simulink model "event_based_v1"  (R2018b)
settings: Solver=FixedStepAuto  StartTime=0.0  StopTime=150  FixedStep=0.01  RelTol=1e-3
undefined symbols (not defined in the file or in its folder): theta01, x01, y01
settings Model: Creator=root  LastModifiedBy=root

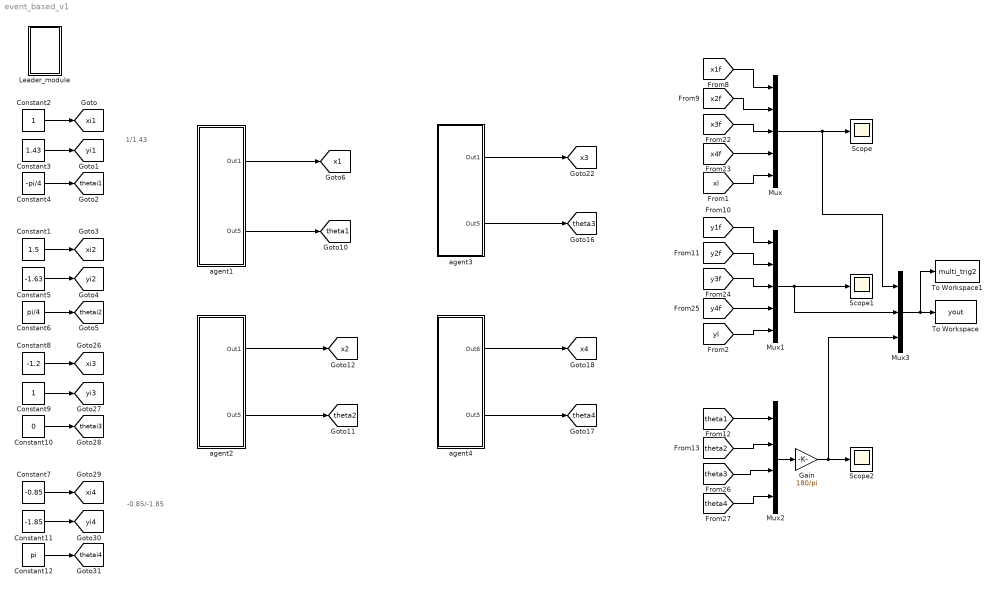
== system event_based_v1 ==
  note: 1/1.43
  note: -0.85/-1.85
  Constant1 : Constant  Value=1.5
  Constant10 : Constant  Value=0
  Constant11 : Constant  Value=-1.85
  Constant12 : Constant  Value=pi
  Constant2 : Constant
  Constant3 : Constant  Value=1.43
  Constant4 : Constant  Value=-pi/4
  Constant5 : Constant  Value=-1.63
  Constant6 : Constant  Value=pi/4
  Constant7 : Constant  Value=-0.85
  Constant8 : Constant  Value=-1.2
  Constant9 : Constant
  Gain : Gain  Gain=180/pi
  Leader_module : Subsystem
  Mux : Mux  Inputs=5
  Mux1 : Mux  Inputs=5
  Mux2 : Mux
  Mux3 : Mux  Inputs=3
  Scope : Scope
  Scope1 : Scope
  Scope2 : Scope
  To Workspace : ToWorkspace  VariableName=yout  SampleTime=-1
      settings: Save2DSignal=2-D array (concatenate along first dimension)
  To Workspace1 : ToWorkspace  VariableName=multi_trig2  SaveFormat=Structure With Time  SampleTime=-1
  agent1 : Subsystem
  agent2 : Subsystem
  agent3 : Subsystem
  agent4 : Subsystem
  tag scope: theta1=global, theta2=global, theta3=global, theta4=global, thetai1=global, thetai2=global, thetai3=global, thetai4=global, x1=global, x2=global, x3=global, x4=global, xi1=global, xi2=global, xi3=global, xi4=global, yi1=global, yi2=global, yi3=global, yi4=global
  wires:
  Mux3/1 -> To Workspace/1, To Workspace1/1
  Mux2/1 -> Gain/1
  [theta4] -> Mux2/4
  [theta3] -> Mux2/3
  [theta2] -> Mux2/2
  Mux1/1 -> Scope1/1, Mux3/2
  [y4f] -> Mux1/4
  [y3f] -> Mux1/3
  [y2f] -> Mux1/2
  [x4f] -> Mux/4
  [x3f] -> Mux/3
  Constant9/1 -> [yi3]
  Constant10/1 -> [thetai3]
  Constant8/1 -> [xi3]
  Constant7/1 -> [xi4]
  Constant12/1 -> [thetai4]
  Constant11/1 -> [yi4]
  agent3/2(Out5) -> [theta3]
  agent4/2(Out5) -> [theta4]
  Gain/1 -> Scope2/1, Mux3/3
  [theta1] -> Mux2/1
  Mux/1 -> Mux3/1, Scope/1
  [y1f] -> Mux1/1
  [x2f] -> Mux/2
  [x1f] -> Mux/1
  agent2/2(Out5) -> [theta2]
  agent1/2(Out5) -> [theta1]
  Constant5/1 -> [yi2]
  Constant6/1 -> [thetai2]
  Constant1/1 -> [xi2]
  Constant2/1 -> [xi1]
  Constant4/1 -> [thetai1]
  Constant3/1 -> [yi1]
  [xl] -> Mux/5
  [yl] -> Mux1/5
  agent1/1(Out1) -> [x1]
  agent2/1(Out1) -> [x2]
  agent3/1(Out1) -> [x3]
  agent4/1(Out6) -> [x4]

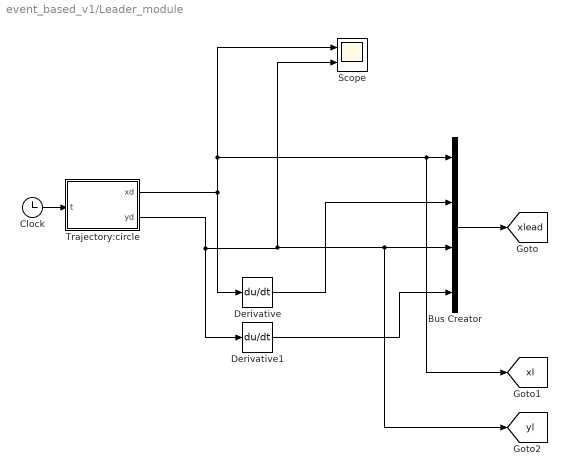
== system event_based_v1/Leader_module ==
  Bus Creator : BusCreator  Inputs=4
  Clock : Clock
  Derivative : Derivative
  Derivative1 : Derivative
  Scope : Scope  NumInputPorts=2
  Trajectory:circle : MATLAB Function  TreatAsAtomicUnit=on
  tag scope: xl=global, xlead=global, yl=global
  wires:
  Trajectory:circle/2(yd) -> [yl], Bus Creator/3, Scope/2, Derivative1/1
  Trajectory:circle/1(xd) -> Scope/1, [xl], Bus Creator/1, Derivative/1
  Clock/1 -> Trajectory:circle/1(t)
  Bus Creator/1 -> [xlead]
  Derivative/1 -> Bus Creator/2
  Derivative1/1 -> Bus Creator/4

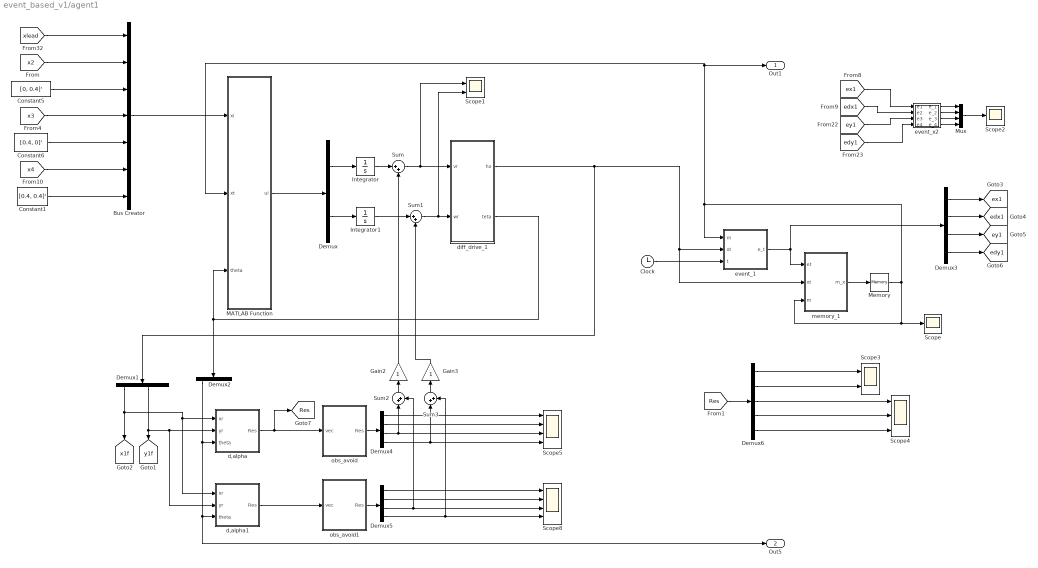
== system event_based_v1/agent1 ==
  Bus Creator : BusCreator  Inputs=7
  Clock : Clock
  Constant1 : Constant  Value=[0.4, 0.4]'
  Constant5 : Constant  Value=[0, 0.4]'
  Constant6 : Constant  Value=[0.4, 0]'
  Demux : Demux  Outputs=2
  Demux{1,3..5} (4 alike) : Demux
  Demux2 : Demux  Outputs=3
  Demux6 : Demux  Outputs=5
  Gain2 : Gain
  Gain3 : Gain
  Integrator : Integrator
  Integrator1 : Integrator
  MATLAB Function : MATLAB Function  TreatAsAtomicUnit=on
  Memory : Memory  InitialCondition=[0 0 0 0]'
  Mux : Mux
  Scope : Scope
  Scope1 : Scope  NumInputPorts=2
  Scope2 : Scope
  Scope3 : Scope  NumInputPorts=2
  Scope4 : Scope  NumInputPorts=3
  Scope5 : Scope  NumInputPorts=4
  Scope8 : Scope  NumInputPorts=4
  Sum{,1..3} (4 alike) : Sum  Inputs=|++
  d,alpha : MATLAB Function  TreatAsAtomicUnit=on
  d,alpha1 : MATLAB Function  TreatAsAtomicUnit=on
  diff_drive_1 : Subsystem  mask{base=0.078, base_error=2.5, radius=0.029, radius_error=6.9, omega_max=260}
      mask prompts: base_error "Base error in percent"; radius_error "Radius error in percent"; omega_max "Wheel Max Velocity"
  event_1 : MATLAB Function  TreatAsAtomicUnit=on
  event_x2 : MATLAB Function  TreatAsAtomicUnit=on
  memory_1 : MATLAB Function  TreatAsAtomicUnit=on
  "obs_avoid " : MATLAB Function  TreatAsAtomicUnit=on
  obs_avoid1 : MATLAB Function  TreatAsAtomicUnit=on
  Out1 : Outport
  Out5 : Outport  Port=2
  tag scope: Res=global, edx1=global, edy1=global, ex1=global, ey1=global, x1f=global, y1f=global
  wires:
  Sum3/1 -> Gain3/1
  Sum2/1 -> Gain2/1
  Gain3/1 -> Sum1/2
  Gain2/1 -> Sum/2
  Integrator1/1 -> Sum1/1
  Sum/1 -> diff_drive_1/1(vr), Scope1/1
  Sum1/1 -> diff_drive_1/2(wr), Scope1/2
  Integrator/1 -> Sum/1
  Demux/1 -> Integrator/1
  MATLAB Function/1(ui) -> Demux/1
  Demux/2 -> Integrator1/1
  Bus Creator/1 -> MATLAB Function/1(xi)
  Constant6/1 -> Bus Creator/5
  [xlead] -> Bus Creator/1
  Constant5/1 -> Bus Creator/3
  Constant1/1 -> Bus Creator/7
  [x2] -> Bus Creator/2
  [x4] -> Bus Creator/6
  [x3] -> Bus Creator/4
  diff_drive_1/2(teta) -> Demux2/1, MATLAB Function/3(theta)
  diff_drive_1/1(hx) -> memory_1/2(xt), event_1/2(xt), Demux1/1
  Demux1/1 -> d,alpha1/1(xr), d,alpha/1(xr), [x1f]
  Demux1/3 -> d,alpha1/2(yr), d,alpha/2(yr), [y1f]
  Demux2/1 -> d,alpha/3(theta), Out5/1, d,alpha1/3(theta)
  event_x2/2(e_2) -> Mux/2
  event_x2/3(e_3) -> Mux/3
  [edx1] -> event_x2/2(e2)
  [edy1] -> event_x2/4(e4)
  event_1/1(e_t) -> Demux3/1, memory_1/1(et)
  Memory/1 -> event_1/1(m), Out1/1, MATLAB Function/2(xt), memory_1/3(m), Scope/1
  [ex1] -> event_x2/1(e1)
  Mux/1 -> Scope2/1
  memory_1/1(m_x) -> Memory/1
  event_x2/1(e_1) -> Mux/1
  [ey1] -> event_x2/3(e3)
  event_x2/4(e_4) -> Mux/4
  Clock/1 -> event_1/3(t)
  Demux3/1 -> [ex1]
  Demux3/2 -> [edx1]
  Demux3/3 -> [ey1]
  Demux3/4 -> [edy1]
  d,alpha/1(Res) -> [Res], "obs_avoid "/1(vec)
  "obs_avoid "/1(Res) -> Demux4/1
  Demux5/2 -> Scope8/2
  Demux4/3 -> Sum2/1, Scope5/3
  obs_avoid1/1(Res) -> Demux5/1
  Demux4/2 -> Scope5/2
  Demux5/4 -> Sum3/2, Scope8/4
  Demux5/3 -> Sum2/2, Scope8/3
  Demux4/4 -> Sum3/1, Scope5/4
  d,alpha1/1(Res) -> obs_avoid1/1(vec)
  Demux5/1 -> Scope8/1
  Demux4/1 -> Scope5/1
  [Res] -> Demux6/1
  Demux6/1 -> Scope3/1
  Demux6/2 -> Scope3/2
  Demux6/3 -> Scope4/1
  Demux6/4 -> Scope4/2
  Demux6/5 -> Scope4/3

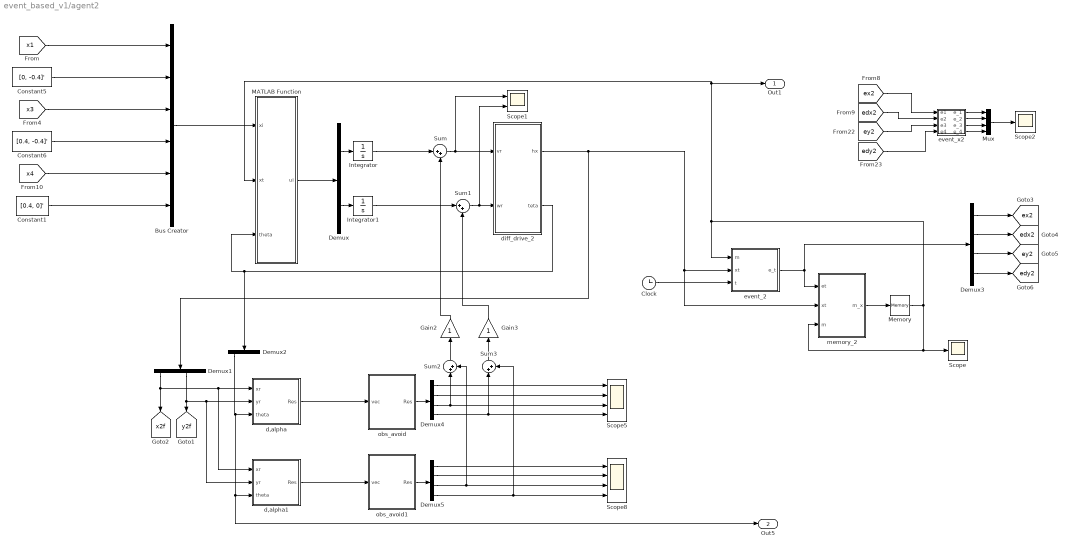
== system event_based_v1/agent2 ==
  Bus Creator : BusCreator  Inputs=6
  Clock : Clock
  Constant1 : Constant  Value=[0.4, 0]'
  Constant5 : Constant  Value=[0, -0.4]'
  Constant6 : Constant  Value=[0.4, -0.4]'
  Demux : Demux  Outputs=2
  Demux{1,3..5} (4 alike) : Demux
  Demux2 : Demux  Outputs=3
  Gain2 : Gain
  Gain3 : Gain
  Integrator : Integrator
  Integrator1 : Integrator
  MATLAB Function : MATLAB Function  TreatAsAtomicUnit=on
  Memory : Memory  InitialCondition=[0 0 0 0]'
  Mux : Mux
  Scope : Scope
  Scope1 : Scope  NumInputPorts=2
  Scope2 : Scope
  Scope5 : Scope  NumInputPorts=4
  Scope8 : Scope  NumInputPorts=4
  Sum{,1..3} (4 alike) : Sum  Inputs=|++
  d,alpha : MATLAB Function  TreatAsAtomicUnit=on
  d,alpha1 : MATLAB Function  TreatAsAtomicUnit=on
  diff_drive_2 : Subsystem  mask{base=0.078, base_error=2.5, radius=0.029, radius_error=6.9, omega_max=260}
      mask prompts: base_error "Base error in percent"; radius_error "Radius error in percent"; omega_max "Wheel Max Velocity"
  event_2 : MATLAB Function  TreatAsAtomicUnit=on
  event_x2 : MATLAB Function  TreatAsAtomicUnit=on
  memory_2 : MATLAB Function  TreatAsAtomicUnit=on
  "obs_avoid " : MATLAB Function  TreatAsAtomicUnit=on
  obs_avoid1 : MATLAB Function  TreatAsAtomicUnit=on
  Out1 : Outport
  Out5 : Outport  Port=2
  tag scope: edx2=global, edy2=global, ex2=global, ey2=global, x2f=global, y2f=global
  wires:
  Sum3/1 -> Gain3/1
  Sum2/1 -> Gain2/1
  Sum/1 -> diff_drive_2/1(vr), Scope1/1
  Gain2/1 -> Sum/2
  Integrator/1 -> Sum/1
  Sum1/1 -> diff_drive_2/2(wr), Scope1/2
  Gain3/1 -> Sum1/2
  Integrator1/1 -> Sum1/1
  diff_drive_2/2(teta) -> Demux2/1, MATLAB Function/3(theta)
  Demux/2 -> Integrator1/1
  MATLAB Function/1(ui) -> Demux/1
  Demux/1 -> Integrator/1
  Bus Creator/1 -> MATLAB Function/1(xi)
  [x1] -> Bus Creator/1
  Constant6/1 -> Bus Creator/4
  Constant5/1 -> Bus Creator/2
  [x3] -> Bus Creator/3
  Constant1/1 -> Bus Creator/6
  [x4] -> Bus Creator/5
  Demux1/1 -> d,alpha/1(xr), d,alpha1/1(xr), [x2f]
  Demux1/3 -> d,alpha/2(yr), d,alpha1/2(yr), [y2f]
  Demux2/1 -> d,alpha/3(theta), d,alpha1/3(theta), Out5/1
  Memory/1 -> Out1/1, MATLAB Function/2(xt), event_2/1(m), memory_2/3(m), Scope/1
  event_2/1(e_t) -> Demux3/1, memory_2/1(et)
  Clock/1 -> event_2/3(t)
  Demux3/4 -> [edy2]
  diff_drive_2/1(hx) -> memory_2/2(xt), event_2/2(xt), Demux1/1
  memory_2/1(m_x) -> Memory/1
  Demux3/1 -> [ex2]
  Demux3/3 -> [ey2]
  Demux3/2 -> [edx2]
  [edy2] -> event_x2/4(e4)
  event_x2/4(e_4) -> Mux/4
  [edx2] -> event_x2/2(e2)
  event_x2/2(e_2) -> Mux/2
  [ex2] -> event_x2/1(e1)
  event_x2/3(e_3) -> Mux/3
  Mux/1 -> Scope2/1
  [ey2] -> event_x2/3(e3)
  event_x2/1(e_1) -> Mux/1
  Demux5/2 -> Scope8/2
  Demux5/4 -> Sum3/2, Scope8/4
  "obs_avoid "/1(Res) -> Demux4/1
  Demux4/2 -> Scope5/2
  d,alpha/1(Res) -> "obs_avoid "/1(vec)
  obs_avoid1/1(Res) -> Demux5/1
  d,alpha1/1(Res) -> obs_avoid1/1(vec)
  Demux5/3 -> Sum2/2, Scope8/3
  Demux4/4 -> Sum3/1, Scope5/4
  Demux5/1 -> Scope8/1
  Demux4/3 -> Scope5/3, Sum2/1
  Demux4/1 -> Scope5/1

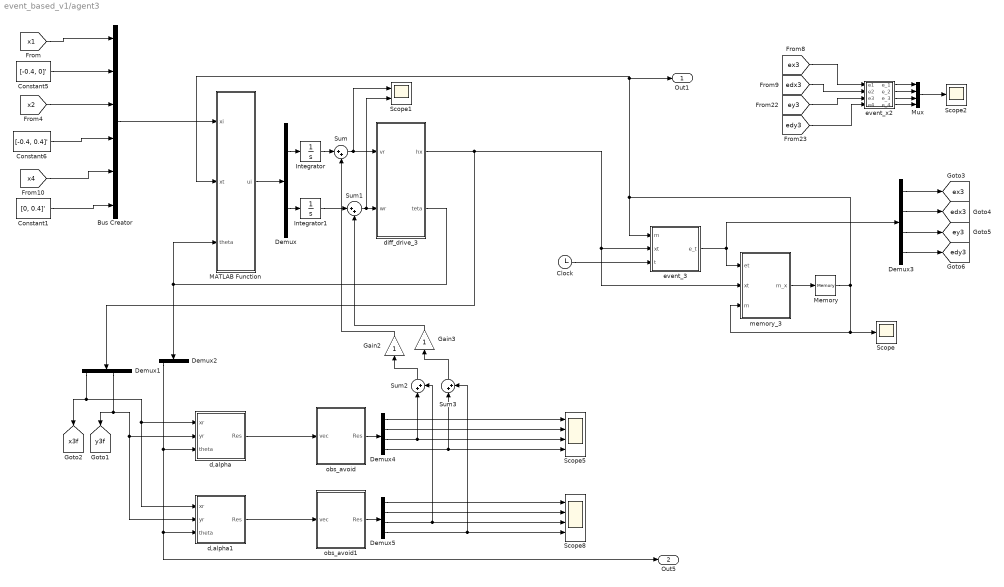
== system event_based_v1/agent3 ==
  Bus Creator : BusCreator  Inputs=6
  Clock : Clock
  Constant1 : Constant  Value=[0, 0.4]'
  Constant5 : Constant  Value=[-0.4, 0]'
  Constant6 : Constant  Value=[-0.4, 0.4]'
  Demux : Demux  Outputs=2
  Demux{1,3..5} (4 alike) : Demux
  Demux2 : Demux  Outputs=3
  Gain2 : Gain
  Gain3 : Gain
  Integrator : Integrator
  Integrator1 : Integrator
  MATLAB Function : MATLAB Function  TreatAsAtomicUnit=on
  Memory : Memory  InitialCondition=[0 0 0 0]'
  Mux : Mux
  Scope : Scope
  Scope1 : Scope  NumInputPorts=2
  Scope2 : Scope
  Scope5 : Scope  NumInputPorts=4
  Scope8 : Scope  NumInputPorts=4
  Sum{,1..3} (4 alike) : Sum  Inputs=|++
  d,alpha : MATLAB Function  TreatAsAtomicUnit=on
  d,alpha1 : MATLAB Function  TreatAsAtomicUnit=on
  "diff_drive_3 " : Subsystem  mask{base=0.078, base_error=2.5, radius=0.029, radius_error=6.9, omega_max=260}
      mask prompts: base_error "Base error in percent"; radius_error "Radius error in percent"; omega_max "Wheel Max Velocity"
  event_3 : MATLAB Function  TreatAsAtomicUnit=on
  event_x2 : MATLAB Function  TreatAsAtomicUnit=on
  memory_3 : MATLAB Function  TreatAsAtomicUnit=on
  "obs_avoid " : MATLAB Function  TreatAsAtomicUnit=on
  obs_avoid1 : MATLAB Function  TreatAsAtomicUnit=on
  Out1 : Outport
  Out5 : Outport  Port=2
  tag scope: edx3=global, edy3=global, ex3=global, ey3=global, x3f=global, y3f=global
  wires:
  Sum3/1 -> Gain3/1
  Sum2/1 -> Gain2/1
  Sum1/1 -> "diff_drive_3 "/2(wr), Scope1/2
  Integrator1/1 -> Sum1/1
  Integrator/1 -> Sum/1
  Sum/1 -> "diff_drive_3 "/1(vr), Scope1/1
  Gain3/1 -> Sum1/2
  Gain2/1 -> Sum/2
  "diff_drive_3 "/2(teta) -> Demux2/1, MATLAB Function/3(theta)
  Demux/2 -> Integrator1/1
  MATLAB Function/1(ui) -> Demux/1
  Demux/1 -> Integrator/1
  Bus Creator/1 -> MATLAB Function/1(xi)
  Constant5/1 -> Bus Creator/2
  [x2] -> Bus Creator/3
  Constant6/1 -> Bus Creator/4
  Constant1/1 -> Bus Creator/6
  [x1] -> Bus Creator/1
  [x4] -> Bus Creator/5
  Demux1/1 -> d,alpha1/1(xr), d,alpha/1(xr), [x3f]
  Demux1/3 -> d,alpha1/2(yr), d,alpha/2(yr), [y3f]
  Demux2/1 -> Out5/1, d,alpha1/3(theta), d,alpha/3(theta)
  Demux3/2 -> [edx3]
  Demux3/1 -> [ex3]
  Mux/1 -> Scope2/1
  memory_3/1(m_x) -> Memory/1
  [ex3] -> event_x2/1(e1)
  Memory/1 -> event_3/1(m), MATLAB Function/2(xt), Out1/1, memory_3/3(m), Scope/1
  [edy3] -> event_x2/4(e4)
  Demux3/4 -> [edy3]
  [ey3] -> event_x2/3(e3)
  Clock/1 -> event_3/3(t)
  event_3/1(e_t) -> Demux3/1, memory_3/1(et)
  event_x2/3(e_3) -> Mux/3
  event_x2/4(e_4) -> Mux/4
  event_x2/2(e_2) -> Mux/2
  [edx3] -> event_x2/2(e2)
  "diff_drive_3 "/1(hx) -> memory_3/2(xt), event_3/2(xt), Demux1/1
  Demux3/3 -> [ey3]
  event_x2/1(e_1) -> Mux/1
  Demux4/3 -> Sum2/1, Scope5/3
  Demux5/3 -> Sum2/2, Scope8/3
  d,alpha/1(Res) -> "obs_avoid "/1(vec)
  Demux5/2 -> Scope8/2
  Demux4/1 -> Scope5/1
  Demux5/4 -> Sum3/2, Scope8/4
  obs_avoid1/1(Res) -> Demux5/1
  Demux4/4 -> Sum3/1, Scope5/4
  Demux5/1 -> Scope8/1
  d,alpha1/1(Res) -> obs_avoid1/1(vec)
  Demux4/2 -> Scope5/2
  "obs_avoid "/1(Res) -> Demux4/1

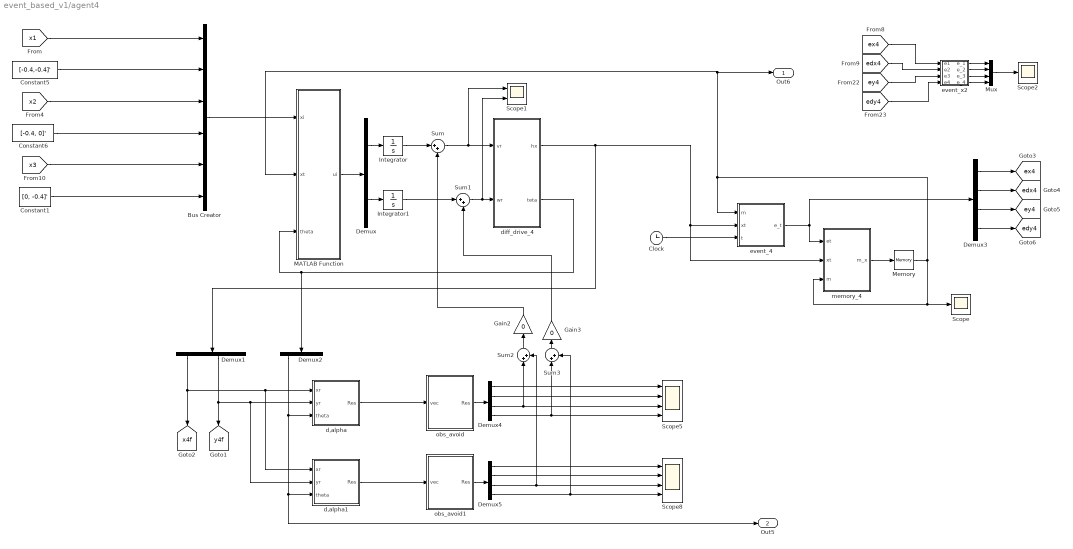
== system event_based_v1/agent4 ==
  Bus Creator : BusCreator  Inputs=6
  Clock : Clock
  Constant1 : Constant  Value=[0, -0.4]'
  Constant5 : Constant  Value=[-0.4,-0.4]'
  Constant6 : Constant  Value=[-0.4, 0]'
  Demux : Demux  Outputs=2
  Demux{1,3..5} (4 alike) : Demux
  Demux2 : Demux  Outputs=3
  Gain2 : Gain  Gain=0
  Gain3 : Gain  Gain=0
  Integrator : Integrator
  Integrator1 : Integrator
  MATLAB Function : MATLAB Function  TreatAsAtomicUnit=on
  Memory : Memory  InitialCondition=[0 0 0 0]'
  Mux : Mux
  Scope : Scope
  Scope1 : Scope  NumInputPorts=2
  Scope2 : Scope
  Scope5 : Scope  NumInputPorts=4
  Scope8 : Scope  NumInputPorts=4
  Sum{,1..3} (4 alike) : Sum  Inputs=|++
  d,alpha : MATLAB Function  TreatAsAtomicUnit=on
  d,alpha1 : MATLAB Function  TreatAsAtomicUnit=on
  diff_drive_4 : Subsystem  mask{base=0.078, base_error=2.5, radius=0.029, radius_error=6.9, omega_max=260}
      mask prompts: base_error "Base error in percent"; radius_error "Radius error in percent"; omega_max "Wheel Max Velocity"
  event_4 : MATLAB Function  TreatAsAtomicUnit=on
  event_x2 : MATLAB Function  TreatAsAtomicUnit=on
  memory_4 : MATLAB Function  TreatAsAtomicUnit=on
  "obs_avoid " : MATLAB Function  TreatAsAtomicUnit=on
  obs_avoid1 : MATLAB Function  TreatAsAtomicUnit=on
  Out6 : Outport
  Out5 : Outport  Port=2
  tag scope: edx4=global, edy4=global, ex4=global, ey4=global, x4f=global, y4f=global
  wires:
  Sum2/1 -> Gain2/1
  Sum3/1 -> Gain3/1
  Integrator1/1 -> Sum1/1
  Gain3/1 -> Sum1/2
  Sum1/1 -> diff_drive_4/2(wr), Scope1/2
  Sum/1 -> diff_drive_4/1(vr), Scope1/1
  Gain2/1 -> Sum/2
  Integrator/1 -> Sum/1
  Demux/1 -> Integrator/1
  MATLAB Function/1(ui) -> Demux/1
  Demux/2 -> Integrator1/1
  diff_drive_4/2(teta) -> MATLAB Function/3(theta), Demux2/1
  Bus Creator/1 -> MATLAB Function/1(xi)
  Constant5/1 -> Bus Creator/2
  Constant6/1 -> Bus Creator/4
  [x1] -> Bus Creator/1
  [x2] -> Bus Creator/3
  [x3] -> Bus Creator/5
  Constant1/1 -> Bus Creator/6
  Demux1/1 -> [x4f], d,alpha1/1(xr), d,alpha/1(xr)
  Demux1/3 -> [y4f], d,alpha1/2(yr), d,alpha/2(yr)
  Demux2/1 -> d,alpha/3(theta), d,alpha1/3(theta), Out5/1
  Demux3/2 -> [edx4]
  Demux3/1 -> [ex4]
  Mux/1 -> Scope2/1
  memory_4/1(m_x) -> Memory/1
  [ex4] -> event_x2/1(e1)
  Memory/1 -> event_4/1(m), MATLAB Function/2(xt), Out6/1, memory_4/3(m), Scope/1
  [edy4] -> event_x2/4(e4)
  Demux3/4 -> [edy4]
  [ey4] -> event_x2/3(e3)
  Clock/1 -> event_4/3(t)
  event_4/1(e_t) -> Demux3/1, memory_4/1(et)
  event_x2/3(e_3) -> Mux/3
  event_x2/4(e_4) -> Mux/4
  event_x2/2(e_2) -> Mux/2
  [edx4] -> event_x2/2(e2)
  diff_drive_4/1(hx) -> memory_4/2(xt), event_4/2(xt), Demux1/1
  Demux3/3 -> [ey4]
  event_x2/1(e_1) -> Mux/1
  d,alpha/1(Res) -> "obs_avoid "/1(vec)
  "obs_avoid "/1(Res) -> Demux4/1
  Demux4/1 -> Scope5/1
  Demux4/2 -> Scope5/2
  Demux4/3 -> Sum2/1, Scope5/3
  Demux4/4 -> Sum3/1, Scope5/4
  d,alpha1/1(Res) -> obs_avoid1/1(vec)
  obs_avoid1/1(Res) -> Demux5/1
  Demux5/4 -> Sum3/2, Scope8/4
  Demux5/3 -> Sum2/2, Scope8/3
  Demux5/2 -> Scope8/2
  Demux5/1 -> Scope8/1

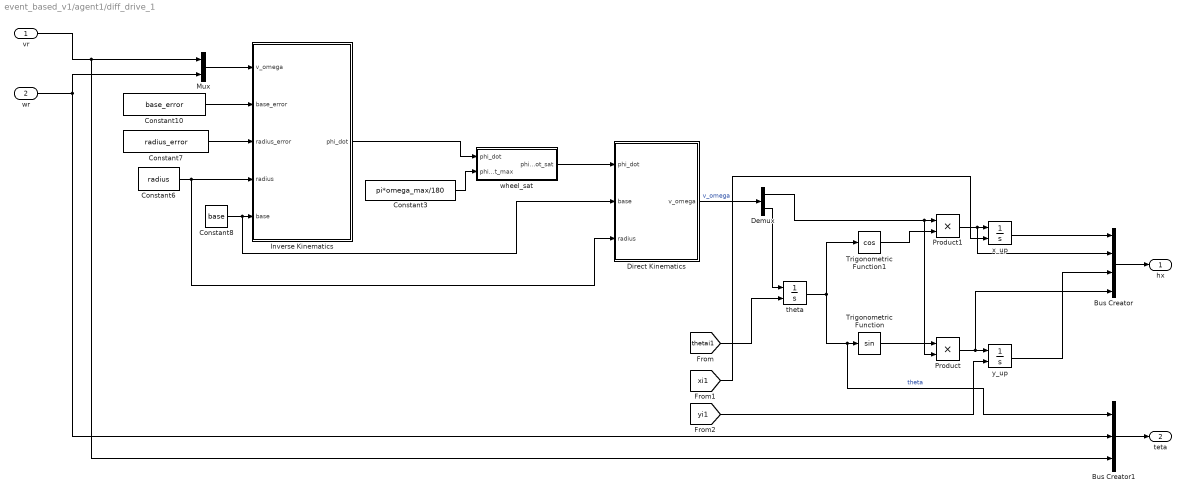
== system event_based_v1/agent1/diff_drive_1 ==
  vr : Inport
  wr : Inport  Port=2
  Bus Creator : BusCreator  Inputs=4
  Bus Creator1 : BusCreator  Inputs=3
  Constant10 : Constant  Value=base_error
  Constant3 : Constant  Value=pi*omega_max/180
  Constant6 : Constant  Value=radius
  Constant7 : Constant  Value=radius_error
  Constant8 : Constant  Value=base
  Demux : Demux  Outputs=2
  Direct Kinematics : MATLAB Function  TreatAsAtomicUnit=on
  Inverse Kinematics : MATLAB Function  TreatAsAtomicUnit=on
  Mux : Mux  Inputs=2
  Product : Product
  Product1 : Product
  Trigonometric Function : Trigonometry
  Trigonometric Function1 : Trigonometry  Operator=cos
  theta : Integrator  InitialConditionSource=external  InitialCondition=theta01
  wheel_sat : Subsystem
  x_up : Integrator  InitialConditionSource=external  InitialCondition=x01
  y_up : Integrator  InitialConditionSource=external  InitialCondition=y01
  hx : Outport
  teta : Outport  Port=2
  wires:
  theta/1 -> Bus Creator1/1, Trigonometric Function/1, Trigonometric Function1/1  "theta"
  Trigonometric Function1/1 -> Product1/2
  Trigonometric Function/1 -> Product/1
  Product/1 -> Bus Creator/4, y_up/1
  Product1/1 -> Bus Creator/2, x_up/1
  Constant3/1 -> wheel_sat/2(phi_dot_max)
  Direct Kinematics/1(v_omega) -> Demux/1  "v_omega"
  Demux/1 -> Product/2, Product1/1
  Demux/2 -> theta/1
  wheel_sat/1(phi_dot_sat) -> Direct Kinematics/1(phi_dot)
  Inverse Kinematics/1(phi_dot) -> wheel_sat/1(phi_dot)
  Constant10/1 -> Inverse Kinematics/2(base_error)
  Constant7/1 -> Inverse Kinematics/3(radius_error)
  Constant6/1 -> Inverse Kinematics/4(radius), Direct Kinematics/3(radius)
  Constant8/1 -> Direct Kinematics/2(base), Inverse Kinematics/5(base)
  wr/1 -> Bus Creator1/2, Mux/2
  vr/1 -> Bus Creator1/3, Mux/1
  Mux/1 -> Inverse Kinematics/1(v_omega)
  y_up/1 -> Bus Creator/3
  [thetai1] -> theta/2
  [xi1] -> x_up/2
  [yi1] -> y_up/2
  Bus Creator/1 -> hx/1
  x_up/1 -> Bus Creator/1
  Bus Creator1/1 -> teta/1

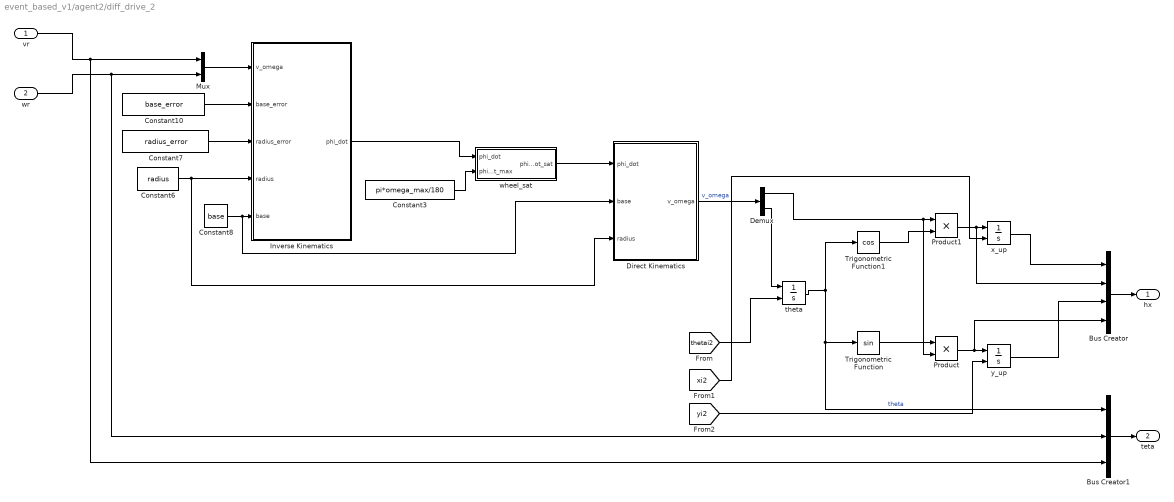
== system event_based_v1/agent2/diff_drive_2 ==
  vr : Inport
  wr : Inport  Port=2
  Bus Creator : BusCreator  Inputs=4
  Bus Creator1 : BusCreator  Inputs=3
  Constant10 : Constant  Value=base_error
  Constant3 : Constant  Value=pi*omega_max/180
  Constant6 : Constant  Value=radius
  Constant7 : Constant  Value=radius_error
  Constant8 : Constant  Value=base
  Demux : Demux  Outputs=2
  Direct Kinematics : MATLAB Function  TreatAsAtomicUnit=on
  Inverse Kinematics : MATLAB Function  TreatAsAtomicUnit=on
  Mux : Mux  Inputs=2
  Product : Product
  Product1 : Product
  Trigonometric Function : Trigonometry
  Trigonometric Function1 : Trigonometry  Operator=cos
  theta : Integrator  InitialConditionSource=external  InitialCondition=theta01
  wheel_sat : Subsystem
  x_up : Integrator  InitialConditionSource=external  InitialCondition=x01
  y_up : Integrator  InitialConditionSource=external  InitialCondition=y01
  hx : Outport
  teta : Outport  Port=2
  wires:
  theta/1 -> Trigonometric Function1/1, Bus Creator1/1, Trigonometric Function/1  "theta"
  Trigonometric Function1/1 -> Product1/2
  Trigonometric Function/1 -> Product/1
  Product/1 -> Bus Creator/4, y_up/1
  Product1/1 -> Bus Creator/2, x_up/1
  Constant3/1 -> wheel_sat/2(phi_dot_max)
  Direct Kinematics/1(v_omega) -> Demux/1  "v_omega"
  Demux/1 -> Product/2, Product1/1
  Demux/2 -> theta/1
  wheel_sat/1(phi_dot_sat) -> Direct Kinematics/1(phi_dot)
  Inverse Kinematics/1(phi_dot) -> wheel_sat/1(phi_dot)
  Constant10/1 -> Inverse Kinematics/2(base_error)
  Constant7/1 -> Inverse Kinematics/3(radius_error)
  Constant6/1 -> Inverse Kinematics/4(radius), Direct Kinematics/3(radius)
  Constant8/1 -> Direct Kinematics/2(base), Inverse Kinematics/5(base)
  wr/1 -> Bus Creator1/2, Mux/2
  vr/1 -> Bus Creator1/3, Mux/1
  Mux/1 -> Inverse Kinematics/1(v_omega)
  x_up/1 -> Bus Creator/1
  y_up/1 -> Bus Creator/3
  [thetai2] -> theta/2
  [xi2] -> x_up/2
  [yi2] -> y_up/2
  Bus Creator/1 -> hx/1
  Bus Creator1/1 -> teta/1

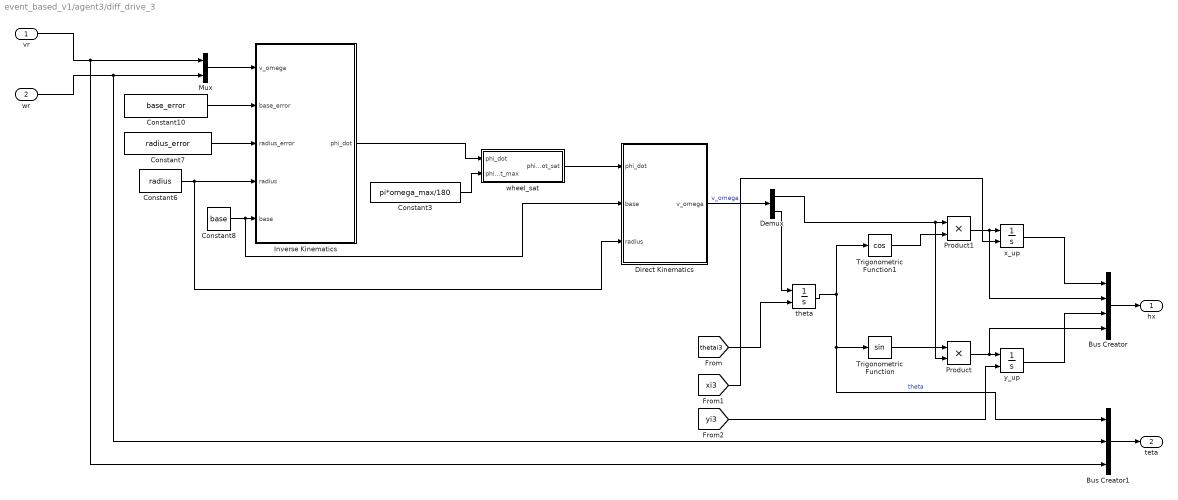
== system event_based_v1/agent3/diff_drive_3  ==
  vr : Inport
  wr : Inport  Port=2
  Bus Creator : BusCreator  Inputs=4
  Bus Creator1 : BusCreator  Inputs=3
  Constant10 : Constant  Value=base_error
  Constant3 : Constant  Value=pi*omega_max/180
  Constant6 : Constant  Value=radius
  Constant7 : Constant  Value=radius_error
  Constant8 : Constant  Value=base
  Demux : Demux  Outputs=2
  Direct Kinematics : MATLAB Function  TreatAsAtomicUnit=on
  Inverse Kinematics : MATLAB Function  TreatAsAtomicUnit=on
  Mux : Mux  Inputs=2
  Product : Product
  Product1 : Product
  Trigonometric Function : Trigonometry
  Trigonometric Function1 : Trigonometry  Operator=cos
  theta : Integrator  InitialConditionSource=external  InitialCondition=theta01
  wheel_sat : Subsystem
  x_up : Integrator  InitialConditionSource=external  InitialCondition=x01
  y_up : Integrator  InitialConditionSource=external  InitialCondition=y01
  hx : Outport
  teta : Outport  Port=2
  wires:
  theta/1 -> Trigonometric Function1/1, Trigonometric Function/1, Bus Creator1/1  "theta"
  Trigonometric Function1/1 -> Product1/2
  Trigonometric Function/1 -> Product/1
  Product/1 -> Bus Creator/4, y_up/1
  Product1/1 -> Bus Creator/2, x_up/1
  Constant3/1 -> wheel_sat/2(phi_dot_max)
  Direct Kinematics/1(v_omega) -> Demux/1  "v_omega"
  Demux/1 -> Product/2, Product1/1
  Demux/2 -> theta/1
  wheel_sat/1(phi_dot_sat) -> Direct Kinematics/1(phi_dot)
  Inverse Kinematics/1(phi_dot) -> wheel_sat/1(phi_dot)
  Constant10/1 -> Inverse Kinematics/2(base_error)
  Constant7/1 -> Inverse Kinematics/3(radius_error)
  Constant6/1 -> Inverse Kinematics/4(radius), Direct Kinematics/3(radius)
  Constant8/1 -> Direct Kinematics/2(base), Inverse Kinematics/5(base)
  wr/1 -> Bus Creator1/2, Mux/2
  vr/1 -> Bus Creator1/3, Mux/1
  Mux/1 -> Inverse Kinematics/1(v_omega)
  [thetai3] -> theta/2
  [xi3] -> x_up/2
  [yi3] -> y_up/2
  Bus Creator/1 -> hx/1
  x_up/1 -> Bus Creator/1
  y_up/1 -> Bus Creator/3
  Bus Creator1/1 -> teta/1

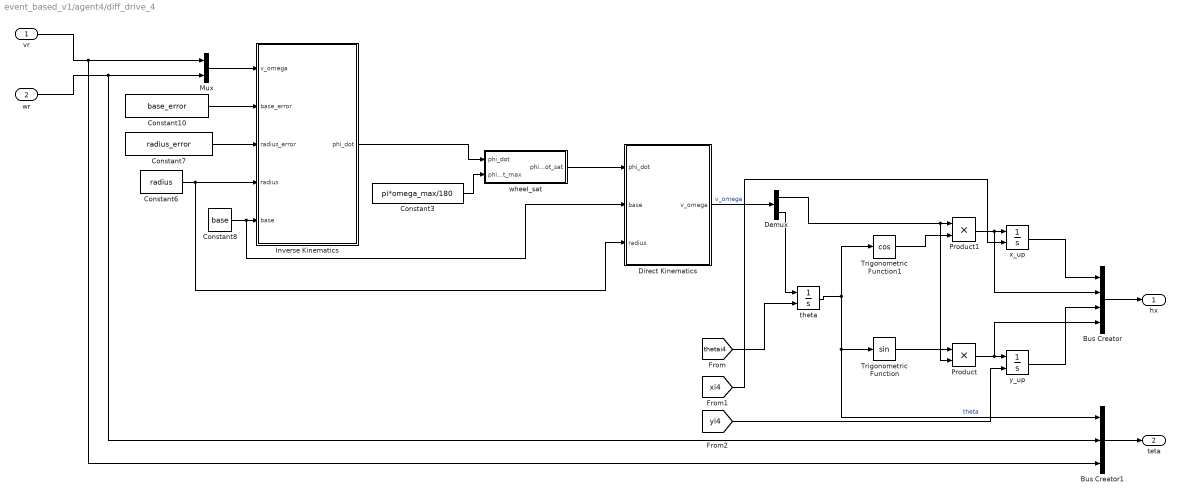
== system event_based_v1/agent4/diff_drive_4 ==
  vr : Inport
  wr : Inport  Port=2
  Bus Creator : BusCreator  Inputs=4
  Bus Creator1 : BusCreator  Inputs=3
  Constant10 : Constant  Value=base_error
  Constant3 : Constant  Value=pi*omega_max/180
  Constant6 : Constant  Value=radius
  Constant7 : Constant  Value=radius_error
  Constant8 : Constant  Value=base
  Demux : Demux  Outputs=2
  Direct Kinematics : MATLAB Function  TreatAsAtomicUnit=on
  Inverse Kinematics : MATLAB Function  TreatAsAtomicUnit=on
  Mux : Mux  Inputs=2
  Product : Product
  Product1 : Product
  Trigonometric Function : Trigonometry
  Trigonometric Function1 : Trigonometry  Operator=cos
  theta : Integrator  InitialConditionSource=external  InitialCondition=theta01
  wheel_sat : Subsystem
  x_up : Integrator  InitialConditionSource=external  InitialCondition=x01
  y_up : Integrator  InitialConditionSource=external  InitialCondition=y01
  hx : Outport
  teta : Outport  Port=2
  wires:
  theta/1 -> Trigonometric Function1/1, Bus Creator1/1, Trigonometric Function/1  "theta"
  Trigonometric Function1/1 -> Product1/2
  Trigonometric Function/1 -> Product/1
  Product/1 -> Bus Creator/4, y_up/1
  Product1/1 -> Bus Creator/2, x_up/1
  Constant3/1 -> wheel_sat/2(phi_dot_max)
  Direct Kinematics/1(v_omega) -> Demux/1  "v_omega"
  Demux/1 -> Product/2, Product1/1
  Demux/2 -> theta/1
  wheel_sat/1(phi_dot_sat) -> Direct Kinematics/1(phi_dot)
  Inverse Kinematics/1(phi_dot) -> wheel_sat/1(phi_dot)
  Constant10/1 -> Inverse Kinematics/2(base_error)
  Constant7/1 -> Inverse Kinematics/3(radius_error)
  Constant6/1 -> Inverse Kinematics/4(radius), Direct Kinematics/3(radius)
  Constant8/1 -> Direct Kinematics/2(base), Inverse Kinematics/5(base)
  wr/1 -> Bus Creator1/2, Mux/2
  vr/1 -> Bus Creator1/3, Mux/1
  Mux/1 -> Inverse Kinematics/1(v_omega)
  [thetai4] -> theta/2
  [xi4] -> x_up/2
  [yi4] -> y_up/2
  Bus Creator/1 -> hx/1
  x_up/1 -> Bus Creator/1
  y_up/1 -> Bus Creator/3
  Bus Creator1/1 -> teta/1

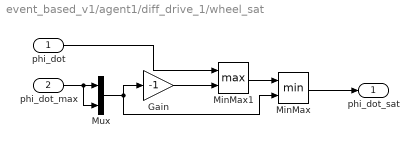
== system event_based_v1/agent1/diff_drive_1/wheel_sat ==
  phi_dot : Inport
  phi_dot_max : Inport  Port=2
  Gain : Gain  Gain=-1
  MinMax : MinMax  Inputs=2
  MinMax1 : MinMax  Function=max  Inputs=2
  Mux : Mux  Inputs=2
  phi_dot_sat : Outport
  wires:
  Gain/1 -> MinMax1/2
  MinMax/1 -> phi_dot_sat/1
  phi_dot_max/1 -> Mux/2, Mux/1
  phi_dot/1 -> MinMax1/1
  MinMax1/1 -> MinMax/1
  Mux/1 -> MinMax/2, Gain/1

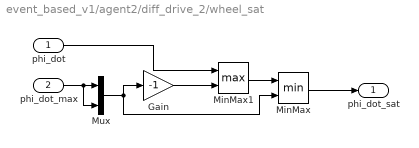
== system event_based_v1/agent2/diff_drive_2/wheel_sat ==
  phi_dot : Inport
  phi_dot_max : Inport  Port=2
  Gain : Gain  Gain=-1
  MinMax : MinMax  Inputs=2
  MinMax1 : MinMax  Function=max  Inputs=2
  Mux : Mux  Inputs=2
  phi_dot_sat : Outport
  wires:
  Gain/1 -> MinMax1/2
  MinMax/1 -> phi_dot_sat/1
  phi_dot_max/1 -> Mux/2, Mux/1
  phi_dot/1 -> MinMax1/1
  MinMax1/1 -> MinMax/1
  Mux/1 -> MinMax/2, Gain/1

== system event_based_v1/agent3/diff_drive_3 /wheel_sat ==
  phi_dot : Inport
  phi_dot_max : Inport  Port=2
  Gain : Gain  Gain=-1
  MinMax : MinMax  Inputs=2
  MinMax1 : MinMax  Function=max  Inputs=2
  Mux : Mux  Inputs=2
  phi_dot_sat : Outport
  wires:
  Gain/1 -> MinMax1/2
  MinMax/1 -> phi_dot_sat/1
  phi_dot_max/1 -> Mux/2, Mux/1
  phi_dot/1 -> MinMax1/1
  MinMax1/1 -> MinMax/1
  Mux/1 -> MinMax/2, Gain/1

== system event_based_v1/agent4/diff_drive_4/wheel_sat ==
  phi_dot : Inport
  phi_dot_max : Inport  Port=2
  Gain : Gain  Gain=-1
  MinMax : MinMax  Inputs=2
  MinMax1 : MinMax  Function=max  Inputs=2
  Mux : Mux  Inputs=2
  phi_dot_sat : Outport
  wires:
  Gain/1 -> MinMax1/2
  MinMax/1 -> phi_dot_sat/1
  phi_dot_max/1 -> Mux/2, Mux/1
  phi_dot/1 -> MinMax1/1
  MinMax1/1 -> MinMax/1
  Mux/1 -> MinMax/2, Gain/1

== matlab function event_based_v1/agent2/MATLAB Function ==
  data: xi input; xt input; theta input; ui output
function ui = fcn(xi, xt, theta)

li = 0.01;
kpx = 0.07;
kdx = 0.96;
kpy = 0.07;
kdy = 0.96;

%Extract data from neighbors vector
x1 = xi(1);
dx1 = xi(2);
y1 = xi(3);
dy1 = xi(4);
biasx1 = xi(5);
biasy1 = xi(6);
x3 = xi(7);
dx3 = xi(8);
y3 = xi(9);
dy3 = xi(10);
biasx3 = xi(11);
biasy3 = xi(12);
x4 = xi(13);
dx4 = xi(14);
y4 = xi(15);
dy4 = xi(16);
biasx4 = xi(17);
biasy4 = xi(18);

%Extract data from positions vector
x = xt(1);
dx = xt(2);
y = xt(3);
dy = xt(4);

%Extract data from orientation data vector
the = theta(1);
dthe = theta(2);
vi = theta(3);

A = [cos(the) -li*sin(the); 
     sin(the) li*cos(the)];
 
oex = kpx*(x1 - x + biasx1)+kdx*(dx1-dx);
oey = kpy*(y1 - y + biasy1)+kdy*(dy1-dy);

thex = kpx*(x3 - x + biasx3)+kdx*(dx3-dx);
they = kpy*(y3 - y + biasy3)+kdy*(dy3-dy);

fex = kpx*(x4 - x + biasx4)+kdx*(dx4-dx);
fey = kpy*(y4 - y + biasy4)+kdy*(dy4-dy);
 
B = [oex+thex+fex+vi*sin(the)*dthe+dthe^2*li*cos(the);
     oey+they+fey-vi*dthe*cos(the)+dthe^2*li*sin(the)];
 
ui = A\B;

== matlab function event_based_v1/agent1/MATLAB Function ==
  data: xi input; xt input; theta input; ui output
function ui = fcn(xi, xt, theta)

%offest and internal controller parameters
li = 0.01;
kpx = 0.07; %0.07
kdx = 0.96;
kpy = 0.07;
kdy = 0.96;

%Extract data from the vector
xl = xi(1);
dxl = xi(2);
yl = xi(3);
dyl = xi(4);
x2 = xi(5);
dx2 = xi(6);
y2 = xi(7);
dy2 = xi(8);
biasx2 = xi(9);
biasy2 = xi(10);
x3 = xi(11);
dx3 = xi(12);
y3 = xi(13);
dy3 = xi(14);
biasx3 = xi(15);
biasy3 = xi(16);
x4 = xi(17);
dx4 = xi(18);
y4 = xi(19);
dy4 = xi(20);
biasx4 = xi(21);
biasy4 = xi(22);

%Extract data from positions vector
x = xt(1);
dx = xt(2);
y = xt(3);
dy = xt(4);

%Extract data from orientation data vector
the = theta(1);
dthe = theta(2);
vi = theta(3);


A = [cos(the) -li*sin(the); 
     sin(the) li*cos(the)];
 
lex = kpx*(xl - x)+kdx*(dxl-dx);
ley = kpy*(yl - y)+kdy*(dyl-dy);

tex = kpx*(x2 - x + biasx2)+kdx*(dx2-dx);
tey = kpy*(y2 - y + biasy2)+kdy*(dy2-dy);

thex = kpx*(x3 - x + biasx3)+kdx*(dx3-dx);
they = kpy*(y3 - y + biasy3)+kdy*(dy3-dy);

fex = kpx*(x4 - x + biasx4)+kdx*(dx4-dx);
fey = kpy*(y4 - y + biasy4)+kdy*(dy4-dy);
 
B = [lex+tex+thex+fex+vi*sin(the)*dthe+dthe^2*li*cos(the);
     ley+tey+they+fey-vi*dthe*cos(the)+dthe^2*li*sin(the)];
 
ui = A\B;

== matlab function event_based_v1/agent1/d,alpha ==
  data: Res output; xr input; yr input; theta input
function Res = circle(xr, yr, theta)

%%POsition and orientation to the obstacles
obs = atan2(-0.1-yr, 0.8-xr);

alpha = obs - theta;

%%Detection and orientation (left/right) of the object
betal = (pi/2) - alpha;

betar = -(pi/2) - alpha;

dis = sqrt((0.8-xr)^2+(-0.1-yr)^2);

%%We define if the object is to the left or right of the vehicle
if alpha > 0
    dl = dis;
else
    dl = NaN;
end

if alpha <= 0
    dr = dis;
else
    dr = NaN;
end

Res = [betal;betar;dl;dr;dis];

== matlab function event_based_v1/agent2/d,alpha ==
  data: Res output; xr input; yr input; theta input
function Res = circle(xr, yr, theta)

%%POsition and orientation to the obstacles
obs = atan2(-0.1-yr, 0.8-xr);

alpha = obs - theta;

%%Detection and orientation (left/right) of the object
betal = (pi/2) - alpha;

betar = -(pi/2) - alpha;

dis = sqrt((0.8-xr)^2+(-0.1-yr)^2);

%%We define if the object is to the left or right of the vehicle
if alpha > 0
    dl = dis;
else
    dl = NaN;
end

if alpha <= 0
    dr = dis;
else
    dr = NaN;
end

Res = [betal;betar;dl;dr;dis];

== matlab function event_based_v1/agent2/d,alpha1 ==
  data: Res output; xr input; yr input; theta input
function Res = circle(xr, yr, theta)

%%POsition and orientation to the obstacles
obs = atan2(-0.1-yr, 0.9-xr);

alpha = obs - theta;

%%Detection and orientation (left/right) of the object
betal = (pi/2) - alpha;

betar = -(pi/2) - alpha;

dis = sqrt((0.9-xr)^2+(-0.1-yr)^2);

%%We define if the object is to the left or right of the vehicle
if alpha > 0
    dl = dis;
else
    dl = NaN;
end

if alpha <= 0
    dr = dis;
else
    dr = NaN;
end

Res = [betal;betar;dl;dr;dis];

== matlab function event_based_v1/agent3/d,alpha ==
  data: Res output; xr input; yr input; theta input
function Res = circle(xr, yr, theta)

%%POsition and orientation to the obstacles
obs = atan2(-0.1-yr, 0.8-xr);

alpha = obs - theta;

%%Detection and orientation (left/right) of the object
betal = (pi/2) - alpha;

betar = -(pi/2) - alpha;

dis = sqrt((0.8-xr)^2+(-0.1-yr)^2);

%%We define if the object is to the left or right of the vehicle
if alpha > 0
    dl = dis;
else
    dl = NaN;
end

if alpha <= 0
    dr = dis;
else
    dr = NaN;
end

Res = [betal;betar;dl;dr;dis];

== matlab function event_based_v1/agent3/d,alpha1 ==
  data: Res output; xr input; yr input; theta input
function Res = circle(xr, yr, theta)

%%POsition and orientation to the obstacles
obs = atan2(-0.1-yr, 0.9-xr);

alpha = obs - theta;

%%Detection and orientation (left/right) of the object
betal = (pi/2) - alpha;

betar = -(pi/2) - alpha;

dis = sqrt((0.9-xr)^2+(-0.1-yr)^2);

%%We define if the object is to the left or right of the vehicle
if alpha > 0
    dl = dis;
else
    dl = NaN;
end

if alpha <= 0
    dr = dis;
else
    dr = NaN;
end

Res = [betal;betar;dl;dr;dis];

== matlab function event_based_v1/agent4/obs_avoid  ==
  data: vec input; Res output
function Res = data(vec)

%Vector with betas
betal = vec(1);
betar = vec(2);
dl = vec(3);
dr = vec(4);

Fmax = 15;
dmax = 0.25;
dmin = 0.15;
s = 0.5;

I = 1;
B = 0.8;
K = 0.4;

c = Fmax/(dmax - dmin)^2;

if dl < dmax
    Fl = c*(dmax - dl)^2;
    if Fl > Fmax
        Fl = Fmax;
    end  
else
    Fl = 0;
end

if dr < dmax
    Fr = c*(dmax - dr)^2;
    if Fr > Fmax
        Fr = Fmax;
    end  
else
    Fr = 0;
end
   
zi = 1 / (I*s^2 + B*s + K);

Vc = zi * (Fr*sin(betar) - Fl*sin(betal));

wc = zi * (Fr-Fl);

Res = [Fl;Fr;Vc;wc];

== matlab function event_based_v1/agent4/obs_avoid1 ==
  data: vec input; Res output
function Res = data(vec)

%Vector with betas
betal = vec(1);
betar = vec(2);
dl = vec(3);
dr = vec(4);

Fmax = 15;
dmax = 0.25;
dmin = 0.15;
s = 0.5;

I = 1;
B = 0.8;
K = 0.4;

c = Fmax/(dmax - dmin)^2;

if dl < dmax
    Fl = c*(dmax - dl)^2;
    if Fl > Fmax
        Fl = Fmax;
    end  
else
    Fl = 0;
end

if dr < dmax
    Fr = c*(dmax - dr)^2;
    if Fr > Fmax
        Fr = Fmax;
    end  
else
    Fr = 0;
end
   
zi = 1 / (I*s^2 + B*s + K);

Vc = zi * (Fr*sin(betar) - Fl*sin(betal));

wc = zi * (Fr-Fl);

Res = [Fl;Fr;Vc;wc];

== matlab function event_based_v1/agent2/event_2 ==
  data: m input; e_t output; xt input; t input
function e_t = fcn(m, xt, t)

%Vector of memories
m1 = m(1);
m2 = m(2);
m3 = m(3);
m4 = m(4);

%Vector of states
x = xt(1);
dx = xt(2);
y = xt(3);
dy = xt(4);

c0 = 0.022;
c1 = 0;
a = 0.5;
u = 6.5;

ex = [m1-x;u*(m2-dx)];

e_x = abs(ex(1))-(c0+c1*exp(-a*t));
e_dx = abs(ex(2))-(c0+c1*exp(-a*t));

ey = [m3-y;u*(m4-dy)];

e_y = abs(ey(1))-(c0+c1*exp(-a*t));
e_dy = abs(ey(2))-(c0+c1*exp(-a*t));

e_t = [e_x;e_dx;e_y;e_dy];

== matlab function event_based_v1/agent3/MATLAB Function ==
  data: xi input; xt input; theta input; ui output
function ui = fcn(xi, xt, theta)

li = 0.01;
kpx = 0.07;
kdx = 0.96;
kpy = 0.07;
kdy = 0.96;

%Extract data from the vector
x1 = xi(1);
dx1 = xi(2);
y1 = xi(3);
dy1 = xi(4);
biasx1 = xi(5);
biasy1 = xi(6);
x2 = xi(7);
dx2 = xi(8);
y2 = xi(9);
dy2 = xi(10);
biasx2 = xi(11);
biasy2 = xi(12);
x4 = xi(13);
dx4 = xi(14);
y4 = xi(15);
dy4 = xi(16);
biasx4 = xi(17);
biasy4 = xi(18);

%Extract data from positions vector
x = xt(1);
dx = xt(2);
y = xt(3);
dy = xt(4);

%Extract data from orientation data vector
the = theta(1);
dthe = theta(2);
vi = theta(3);

A = [cos(the) -li*sin(the); 
     sin(the) li*cos(the)];
 
oex = kpx*(x1 - x + biasx1)+kdx*(dx1-dx);
oey = kpy*(y1 - y + biasy1)+kdy*(dy1-dy);

tex = kpx*(x2 - x + biasx2)+kdx*(dx2-dx);
tey = kpy*(y2 - y + biasy2)+kdy*(dy2-dy);

fex = kpx*(x4 - x + biasx4)+kdx*(dx4-dx);
fey = kpy*(y4 - y + biasy4)+kdy*(dy4-dy);
 
B = [oex+tex+fex+vi*sin(the)*dthe+dthe^2*li*cos(the);
     oey+tey+fey-vi*dthe*cos(the)+dthe^2*li*sin(the)];
 
ui = A\B;

== matlab function event_based_v1/agent2/memory_2 ==
  data: et input; xt input; m_x output; m input
function m_x = fcn(et, xt, m)

%Vector of threshold
epx = et(1);
edx = et(2);
epy = et(3);
edy = et(4);

%Vector of memories
m_px = m(1);
m_sx = m(2);
m_py = m(3);
m_sy = m(4);

%Vector of states
x = xt(1);
dx = xt(2);
y = xt(3);
dy = xt(4);

if epx > 0
    m_px = x;
else
    m_px = m_px;
end

if edx > 0
    m_dx = dx;
else
    m_dx = m_sx;
end

if epy > 0
    m_py = y;
else
    m_py = m_py;
end

if edy > 0
    m_dy = dy;
else
    m_dy = m_sy;
end

m_x = [m_px;m_dx;m_py;m_dy];

== matlab function event_based_v1/agent2/event_x2 ==
  data: e_1 output; e_2 output; e1 input; e2 input; e3 input; e4 input; e_3 output; e_4 output
function [e_1,e_2, e_3, e_4]  = fcn(e1, e2, e3, e4)

if e1 > 0
    e_1 = 1;
else 
    e_1 = 0;
end

if e2 > 0
    e_2 = 1;
else 
    e_2 = 0;
end

if e3 > 0
    e_3 = 1;
else 
    e_3 = 0;
end

if e4 > 0
    e_4 = 1;
else 
    e_4 = 0;
end

== matlab function event_based_v1/agent3/event_3 ==
  data: m input; e_t output; xt input; t input
function e_t = fcn(m, xt, t)

%Vector of memories
m1 = m(1);
m2 = m(2);
m3 = m(3);
m4 = m(4);

%Vector of states
x = xt(1);
dx = xt(2);
y = xt(3);
dy = xt(4);

c0 = 0.022;
c1 = 0;
a = 0.5;
u = 6.5;

ex = [m1-x;u*(m2-dx)];

e_x = abs(ex(1))-(c0+c1*exp(-a*t));
e_dx = abs(ex(2))-(c0+c1*exp(-a*t));

ey = [m3-y;u*(m4-dy)];

e_y = abs(ey(1))-(c0+c1*exp(-a*t));
e_dy = abs(ey(2))-(c0+c1*exp(-a*t));

e_t = [e_x;e_dx;e_y;e_dy];

== matlab function event_based_v1/agent3/event_x2 ==
  data: e_1 output; e_2 output; e1 input; e2 input; e3 input; e4 input; e_3 output; e_4 output
function [e_1,e_2, e_3, e_4]  = fcn(e1, e2, e3, e4)

if e1 > 0
    e_1 = 1;
else 
    e_1 = 0;
end

if e2 > 0
    e_2 = 1;
else 
    e_2 = 0;
end

if e3 > 0
    e_3 = 1;
else 
    e_3 = 0;
end

if e4 > 0
    e_4 = 1;
else 
    e_4 = 0;
end

== matlab function event_based_v1/agent4/MATLAB Function ==
  data: xi input; xt input; theta input; ui output
function ui = fcn(xi, xt, theta)

li = 0.01;
kpx = 0.07;
kdx = 0.96;
kpy = 0.07;
kdy = 0.96;

%Extract data from the vector
x1 = xi(1);
dx1 = xi(2);
y1 = xi(3);
dy1 = xi(4);
biasx1 = xi(5);
biasy1 = xi(6);
x2 = xi(7);
dx2 = xi(8);
y2 = xi(9);
dy2 = xi(10);
biasx2 = xi(11);
biasy2 = xi(12);
x3 = xi(13);
dx3 = xi(14);
y3 = xi(15);
dy3 = xi(16);
biasx3 = xi(17);
biasy3 = xi(18);

%Extract data from positions vector
x = xt(1);
dx = xt(2);
y = xt(3);
dy = xt(4);

%Extract data from orientation data vector
the = theta(1);
dthe = theta(2);
vi = theta(3);

A = [cos(the) -li*sin(the); 
     sin(the) li*cos(the)];
 
oex = kpx*(x1 - x + biasx1)+kdx*(dx1-dx);
oey = kpy*(y1 - y + biasy1)+kdy*(dy1-dy);

tex = kpx*(x2 - x + biasx2)+kdx*(dx2-dx);
tey = kpy*(y2 - y + biasy2)+kdy*(dy2-dy);

thex = kpx*(x3 - x + biasx3)+kdx*(dx3-dx);
they = kpy*(y3 - y + biasy3)+kdy*(dy3-dy);
 
B = [oex+tex+thex+vi*sin(the)*dthe+dthe^2*li*cos(the);
     oey+tey+they-vi*dthe*cos(the)+dthe^2*li*sin(the)];
 
ui = A\B;

== matlab function event_based_v1/agent1/event_1 ==
  data: m input; e_t output; xt input; t input
function e_t = fcn(m, xt, t)

%Vector of memories
m1 = m(1);
m2 = m(2);
m3 = m(3);
m4 = m(4);

%Vector of states
x = xt(1);
dx = xt(2);
y = xt(3);
dy = xt(4);

c0 = 0.022; %0.04
c1 = 0;
a = 0.5;
u = 6.5;

ex = [m1-x;u*(m2-dx)];

e_x = abs(ex(1))-(c0+c1*exp(-a*t));
e_dx = abs(ex(2))-(c0+c1*exp(-a*t));

ey = [m3-y;u*(m4-dy)];

e_y = abs(ey(1))-(c0+c1*exp(-a*t));
e_dy = abs(ey(2))-(c0+c1*exp(-a*t));

e_t = [e_x;e_dx;e_y;e_dy];

== matlab function event_based_v1/agent3/memory_3 ==
  data: et input; xt input; m_x output; m input
function m_x = fcn(et, xt, m)

%Vector of threshold
epx = et(1);
edx = et(2);
epy = et(3);
edy = et(4);

%Vector of memories
m_px = m(1);
m_sx = m(2);
m_py = m(3);
m_sy = m(4);

%Vector of states
x = xt(1);
dx = xt(2);
y = xt(3);
dy = xt(4);

if epx > 0
    m_px = x;
else
    m_px = m_px;
end

if edx > 0
    m_dx = dx;
else
    m_dx = m_sx;
end

if epy > 0
    m_py = y;
else
    m_py = m_py;
end

if edy > 0
    m_dy = dy;
else
    m_dy = m_sy;
end

m_x = [m_px;m_dx;m_py;m_dy];

== matlab function event_based_v1/agent1/memory_1 ==
  data: et input; xt input; m_x output; m input
function m_x = fcn(et, xt, m)

%Vector of threshold
epx = et(1);
edx = et(2);
epy = et(3);
edy = et(4);

%Vector of memories
m_px = m(1);
m_sx = m(2);
m_py = m(3);
m_sy = m(4);

%Vector of states
x = xt(1);
dx = xt(2);
y = xt(3);
dy = xt(4);

if epx > 0
    m_px = x;
else
    m_px = m_px;
end

if edx > 0
    m_dx = dx;
else
    m_dx = m_sx;
end

if epy > 0
    m_py = y;
else
    m_py = m_py;
end

if edy > 0
    m_dy = dy;
else
    m_dy = m_sy;
end

m_x = [m_px;m_dx;m_py;m_dy];

== matlab function event_based_v1/agent4/event_4 ==
  data: m input; e_t output; xt input; t input
function e_t = fcn(m, xt, t)

%Vector of memories
m1 = m(1);
m2 = m(2);
m3 = m(3);
m4 = m(4);

%Vector of states
x = xt(1);
dx = xt(2);
y = xt(3);
dy = xt(4);

c0 = 0.022;
c1 = 0;
a = 0.5;
u = 6.5;

ex = [m1-x;u*(m2-dx)];

e_x = abs(ex(1))-(c0+c1*exp(-a*t));
e_dx = abs(ex(2))-(c0+c1*exp(-a*t));

ey = [m3-y;u*(m4-dy)];

e_y = abs(ey(1))-(c0+c1*exp(-a*t));
e_dy = abs(ey(2))-(c0+c1*exp(-a*t));

e_t = [e_x;e_dx;e_y;e_dy];

== matlab function event_based_v1/agent4/event_x2 ==
  data: e_1 output; e_2 output; e1 input; e2 input; e3 input; e4 input; e_3 output; e_4 output
function [e_1,e_2, e_3, e_4]  = fcn(e1, e2, e3, e4)

if e1 > 0
    e_1 = 1;
else 
    e_1 = 0;
end

if e2 > 0
    e_2 = 1;
else 
    e_2 = 0;
end

if e3 > 0
    e_3 = 1;
else 
    e_3 = 0;
end

if e4 > 0
    e_4 = 1;
else 
    e_4 = 0;
end

== matlab function event_based_v1/agent4/memory_4 ==
  data: et input; xt input; m_x output; m input
function m_x = fcn(et, xt, m)

%Vector of threshold
epx = et(1);
edx = et(2);
epy = et(3);
edy = et(4);

%Vector of memories
m_px = m(1);
m_sx = m(2);
m_py = m(3);
m_sy = m(4);

%Vector of states
x = xt(1);
dx = xt(2);
y = xt(3);
dy = xt(4);

if epx > 0
    m_px = x;
else
    m_px = m_px;
end

if edx > 0
    m_dx = dx;
else
    m_dx = m_sx;
end

if epy > 0
    m_py = y;
else
    m_py = m_py;
end

if edy > 0
    m_dy = dy;
else
    m_dy = m_sy;
end

m_x = [m_px;m_dx;m_py;m_dy];

== matlab function event_based_v1/agent3/obs_avoid  ==
  data: vec input; Res output
function Res = data(vec)

%Vector with betas
betal = vec(1);
betar = vec(2);
dl = vec(3);
dr = vec(4);

Fmax = 15;
dmax = 0.25;
dmin = 0.15;
s = 0.5;

I = 1;
B = 0.8;
K = 0.4;

c = Fmax/(dmax - dmin)^2;

if dl < dmax
    Fl = c*(dmax - dl)^2;
    if Fl > Fmax
        Fl = Fmax;
    end  
else
    Fl = 0;
end

if dr < dmax
    Fr = c*(dmax - dr)^2;
    if Fr > Fmax
        Fr = Fmax;
    end  
else
    Fr = 0;
end
   
zi = 1 / (I*s^2 + B*s + K);

Vc = zi * (Fr*sin(betar) - Fl*sin(betal));

wc = zi * (Fr-Fl);

Res = [Fl;Fr;Vc;wc];

== matlab function event_based_v1/agent1/event_x2 ==
  data: e_1 output; e_2 output; e1 input; e2 input; e3 input; e4 input; e_3 output; e_4 output
function [e_1,e_2, e_3, e_4]  = fcn(e1, e2, e3, e4)

if e1 > 0
    e_1 = 1;
else 
    e_1 = 0;
end

if e2 > 0
    e_2 = 1;
else 
    e_2 = 0;
end

if e3 > 0
    e_3 = 1;
else 
    e_3 = 0;
end

if e4 > 0
    e_4 = 1;
else 
    e_4 = 0;
end

== matlab function event_based_v1/Leader_module/Trajectory:circle ==
  data: t input; xd output; yd output
function [xd, yd] = circle(t)

x = 1;
y = 1;
r = 1.25;  %1.3


if t<90
    xd = 0;
    yd = 0;
elseif t<150
    xd = 1.6;
    yd = -0.2;
% elseif t<20
%     y = 0.5;   
% elseif t<54
%     y = pos3;     
else
    xd = r * cos(t/30) + x;
    yd = r * sin(t/30) + y;
end

== matlab function event_based_v1/agent1/d,alpha1 ==
  data: Res output; xr input; yr input; theta input
function Res = circle(xr, yr, theta)

%%POsition and orientation to the obstacles
obs = atan2(-0.1-yr, 0.9-xr);

alpha = obs - theta;

%%Detection and orientation (left/right) of the object
betal = (pi/2) - alpha;

betar = -(pi/2) - alpha;

dis = sqrt((0.9-xr)^2+(-0.1-yr)^2);

%%We define if the object is to the left or right of the vehicle
if alpha > 0
    dl = dis;
else
    dl = NaN;
end

if alpha <= 0
    dr = dis;
else
    dr = NaN;
end

Res = [betal;betar;dl;dr;dis];

== matlab function event_based_v1/agent1/obs_avoid  ==
  data: vec input; Res output
function Res = data(vec)

%Vector with betas
betal = vec(1);
betar = vec(2);
dl = vec(3);
dr = vec(4);

Fmax = 15;
dmax = 0.25;
dmin = 0.15;
s = 0.5;

I = 1;
B = 0.8;
K = 0.4;

c = Fmax/(dmax - dmin)^2;

if dl < dmax
    Fl = c*(dmax - dl)^2;
    if Fl > Fmax
        Fl = Fmax;
    end  
else
    Fl = 0;
end

if dr < dmax
    Fr = c*(dmax - dr)^2;
    if Fr > Fmax
        Fr = Fmax;
    end  
else
    Fr = 0;
end
   
zi = 1 / (I*s^2 + B*s + K);

Vc = zi * (Fr*sin(betar) - Fl*sin(betal));

wc = zi * (Fr-Fl);

Res = [Fl;Fr;Vc;wc];

== matlab function event_based_v1/agent2/obs_avoid  ==
  data: vec input; Res output
function Res = data(vec)

%Vector with betas
betal = vec(1);
betar = vec(2);
dl = vec(3);
dr = vec(4);

Fmax = 15;
dmax = 0.25;
dmin = 0.15;
s = 0.5;

I = 1;
B = 0.8;
K = 0.4;

c = Fmax/(dmax - dmin)^2;

if dl < dmax
    Fl = c*(dmax - dl)^2;
    if Fl > Fmax
        Fl = Fmax;
    end  
else
    Fl = 0;
end

if dr < dmax
    Fr = c*(dmax - dr)^2;
    if Fr > Fmax
        Fr = Fmax;
    end  
else
    Fr = 0;
end
   
zi = 1 / (I*s^2 + B*s + K);

Vc = zi * (Fr*sin(betar) - Fl*sin(betal));

wc = zi * (Fr-Fl);

Res = [Fl;Fr;Vc;wc];

== matlab function event_based_v1/agent3/obs_avoid1 ==
  data: vec input; Res output
function Res = data(vec)

%Vector with betas
betal = vec(1);
betar = vec(2);
dl = vec(3);
dr = vec(4);

Fmax = 15;
dmax = 0.25;
dmin = 0.15;
s = 0.5;

I = 1;
B = 0.8;
K = 0.4;

c = Fmax/(dmax - dmin)^2;

if dl < dmax
    Fl = c*(dmax - dl)^2;
    if Fl > Fmax
        Fl = Fmax;
    end  
else
    Fl = 0;
end

if dr < dmax
    Fr = c*(dmax - dr)^2;
    if Fr > Fmax
        Fr = Fmax;
    end  
else
    Fr = 0;
end
   
zi = 1 / (I*s^2 + B*s + K);

Vc = zi * (Fr*sin(betar) - Fl*sin(betal));

wc = zi * (Fr-Fl);

Res = [Fl;Fr;Vc;wc];

== matlab function event_based_v1/agent2/obs_avoid1 ==
  data: vec input; Res output
function Res = data(vec)

%Vector with betas
betal = vec(1);
betar = vec(2);
dl = vec(3);
dr = vec(4);

Fmax = 15;
dmax = 0.25;
dmin = 0.15;
s = 0.5;

I = 1;
B = 0.8;
K = 0.4;

c = Fmax/(dmax - dmin)^2;

if dl < dmax
    Fl = c*(dmax - dl)^2;
    if Fl > Fmax
        Fl = Fmax;
    end  
else
    Fl = 0;
end

if dr < dmax
    Fr = c*(dmax - dr)^2;
    if Fr > Fmax
        Fr = Fmax;
    end  
else
    Fr = 0;
end
   
zi = 1 / (I*s^2 + B*s + K);

Vc = zi * (Fr*sin(betar) - Fl*sin(betal));

wc = zi * (Fr-Fl);

Res = [Fl;Fr;Vc;wc];

== matlab function event_based_v1/agent1/obs_avoid1 ==
  data: vec input; Res output
function Res = data(vec)

%Vector with betas
betal = vec(1);
betar = vec(2);
dl = vec(3);
dr = vec(4);

Fmax = 15;
dmax = 0.25;
dmin = 0.15;
s = 0.5;

I = 1;
B = 0.8;
K = 0.4;

c = Fmax/(dmax - dmin)^2;

if dl < dmax
    Fl = c*(dmax - dl)^2;
    if Fl > Fmax
        Fl = Fmax;
    end  
else
    Fl = 0;
end

if dr < dmax
    Fr = c*(dmax - dr)^2;
    if Fr > Fmax
        Fr = Fmax;
    end  
else
    Fr = 0;
end
   
zi = 1 / (I*s^2 + B*s + K);

Vc = zi * (Fr*sin(betar) - Fl*sin(betal));

wc = zi * (Fr-Fl);

Res = [Fl;Fr;Vc;wc];

== matlab function event_based_v1/agent4/d,alpha ==
  data: Res output; xr input; yr input; theta input
function Res = circle(xr, yr, theta)

%%POsition and orientation to the obstacles
obs = atan2(-0.1-yr, 0.8-xr);

alpha = obs - theta;

%%Detection and orientation (left/right) of the object
betal = (pi/2) - alpha;

betar = -(pi/2) - alpha;

dis = sqrt((0.8-xr)^2+(-0.1-yr)^2);

%%We define if the object is to the left or right of the vehicle
if alpha > 0
    dl = dis;
else
    dl = NaN;
end

if alpha <= 0
    dr = dis;
else
    dr = NaN;
end

Res = [betal;betar;dl;dr;dis];

== matlab function event_based_v1/agent4/d,alpha1 ==
  data: Res output; xr input; yr input; theta input
function Res = circle(xr, yr, theta)

%%POsition and orientation to the obstacles
obs = atan2(-0.1-yr, 0.9-xr);

alpha = obs - theta;

%%Detection and orientation (left/right) of the object
betal = (pi/2) - alpha;

betar = -(pi/2) - alpha;

dis = sqrt((0.9-xr)^2+(-0.1-yr)^2);

%%We define if the object is to the left or right of the vehicle
if alpha > 0
    dl = dis;
else
    dl = NaN;
end

if alpha <= 0
    dr = dis;
else
    dr = NaN;
end

Res = [betal;betar;dl;dr;dis];

== matlab function event_based_v1/agent2/diff_drive_2/Direct Kinematics ==
  data: phi_dot input; v_omega output; base input; radius input
function v_omega = dk(phi_dot, base, radius)

v_omega = [radius*(phi_dot(1)+phi_dot(2))/2; radius*(phi_dot(1)-phi_dot(2))/(2*base)];

== matlab function event_based_v1/agent2/diff_drive_2/Inverse Kinematics ==
  data: v_omega input; base_error input; radius_error input; radius input; phi_dot output; base input
function phi_dot = ik(v_omega, base_error, radius_error, radius, base)

base = base * (1+base_error*0.01);
radius = radius * (1+radius_error*0.01);

phi_dot = [(v_omega(1)+base*v_omega(2))/radius; (v_omega(1)-base*v_omega(2))/radius];

== matlab function event_based_v1/agent1/diff_drive_1/Direct Kinematics ==
  data: phi_dot input; v_omega output; base input; radius input
function v_omega = dk(phi_dot, base, radius)

v_omega = [radius*(phi_dot(1)+phi_dot(2))/2; radius*(phi_dot(1)-phi_dot(2))/(2*base)];

== matlab function event_based_v1/agent1/diff_drive_1/Inverse Kinematics ==
  data: v_omega input; base_error input; radius_error input; radius input; phi_dot output; base input
function phi_dot = ik(v_omega, base_error, radius_error, radius, base)

base = base * (1+base_error*0.01);
radius = radius * (1+radius_error*0.01);

phi_dot = [(v_omega(1)+base*v_omega(2))/radius; (v_omega(1)-base*v_omega(2))/radius];

== matlab function event_based_v1/agent3/diff_drive_3 /Direct Kinematics ==
  data: phi_dot input; v_omega output; base input; radius input
function v_omega = dk(phi_dot, base, radius)

v_omega = [radius*(phi_dot(1)+phi_dot(2))/2; radius*(phi_dot(1)-phi_dot(2))/(2*base)];

== matlab function event_based_v1/agent3/diff_drive_3 /Inverse Kinematics ==
  data: v_omega input; base_error input; radius_error input; radius input; phi_dot output; base input
function phi_dot = ik(v_omega, base_error, radius_error, radius, base)

base = base * (1+base_error*0.01);
radius = radius * (1+radius_error*0.01);

phi_dot = [(v_omega(1)+base*v_omega(2))/radius; (v_omega(1)-base*v_omega(2))/radius];

== matlab function event_based_v1/agent4/diff_drive_4/Direct Kinematics ==
  data: phi_dot input; v_omega output; base input; radius input
function v_omega = dk(phi_dot, base, radius)

v_omega = [radius*(phi_dot(1)+phi_dot(2))/2; radius*(phi_dot(1)-phi_dot(2))/(2*base)];

== matlab function event_based_v1/agent4/diff_drive_4/Inverse Kinematics ==
  data: v_omega input; base_error input; radius_error input; radius input; phi_dot output; base input
function phi_dot = ik(v_omega, base_error, radius_error, radius, base)

base = base * (1+base_error*0.01);
radius = radius * (1+radius_error*0.01);

phi_dot = [(v_omega(1)+base*v_omega(2))/radius; (v_omega(1)-base*v_omega(2))/radius];
